simulink model "mMultipleSubsystems"  (Simulink 7.7)
settings: Solver=FixedStepDiscrete  StartTime=0.0  StopTime=10.0  RelTol=1e-3
PostLoadFcn:
  | assignin('base','compCheck', 0);
InitFcn:
  | evalin('base','compCheck = compCheck + 1;');
CloseFcn:
  | % We are using this to make sure that we do not open/close the referenced model during the ErrorChecking.
  | evalin('base','clear compCheck');
settings Model: Creator=mtocci  LastModifiedBy=mtocci
settings OptimizationCC: InlineParams=on

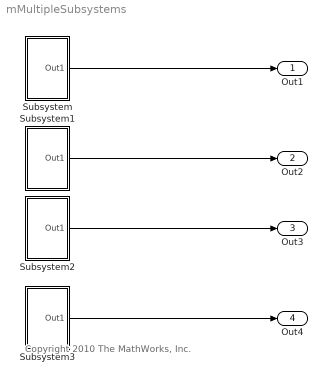
== system mMultipleSubsystems ==
  note: Copyright 2010 The MathWorks, Inc.
  Subsystem : Subsystem  TreatAsAtomicUnit=on
  Subsystem1 : Subsystem  TreatAsAtomicUnit=on
  Subsystem2 : Subsystem  TreatAsAtomicUnit=on
  Subsystem3 : Subsystem  TreatAsAtomicUnit=on
  Out1 : Outport
  Out2 : Outport  Port=2
  Out3 : Outport  Port=3
  Out4 : Outport  Port=4
  wires:
  Subsystem/1(Out1) -> Out1/1
  Subsystem1/1(Out1) -> Out2/1
  Subsystem2/1(Out1) -> Out3/1
  Subsystem3/1(Out1) -> Out4/1

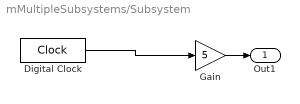
== system mMultipleSubsystems/Subsystem ==
  Digital Clock : DigitalClock
  Gain : Gain  Gain=5
  Out1 : Outport
  wires:
  Digital Clock/1 -> Gain/1
  Gain/1 -> Out1/1

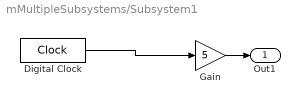
== system mMultipleSubsystems/Subsystem1 ==
  Digital Clock : DigitalClock
  Gain : Gain  Gain=5
  Out1 : Outport
  wires:
  Gain/1 -> Out1/1
  Digital Clock/1 -> Gain/1

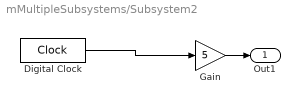
== system mMultipleSubsystems/Subsystem2 ==
  Digital Clock : DigitalClock
  Gain : Gain  Gain=5
  Out1 : Outport
  wires:
  Gain/1 -> Out1/1
  Digital Clock/1 -> Gain/1

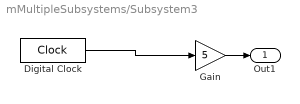
== system mMultipleSubsystems/Subsystem3 ==
  Digital Clock : DigitalClock
  Gain : Gain  Gain=5
  Out1 : Outport
  wires:
  Digital Clock/1 -> Gain/1
  Gain/1 -> Out1/1
